simulink subsystem "quarter_car"  (R2024b)
settings: Solver=VariableStepAuto  StartTime=0.0  StopTime=10.0  RelTol=1e-3
model mask{radius=1, spin_inertia=1, offset=[0; 0; 0], ride_rate=1, damp_rate=0, C_i=0, C_a=0, min_velocity=0, initial_spin=0}
  mask prompts: radius "Wheel radius [m]"; spin_inertia "Wheel inertia [kg m²]"; offset "Resting point offset [m]"; ride_rate "Ride rate [N/m]"; damp_rate "Daming rate [N/(m/s)]"; C_i "Traction coefficient [N]"; C_a "Sideslip coefficient [N]"; min_velocity "Minimum velocity [m/s]"; initial_spin "Initial spin [rad/s]"
libraries: aerolibutil x7, matrix_library x2, simulink x1
settings Model: Creator=yevge  LastModifiedBy=yevge

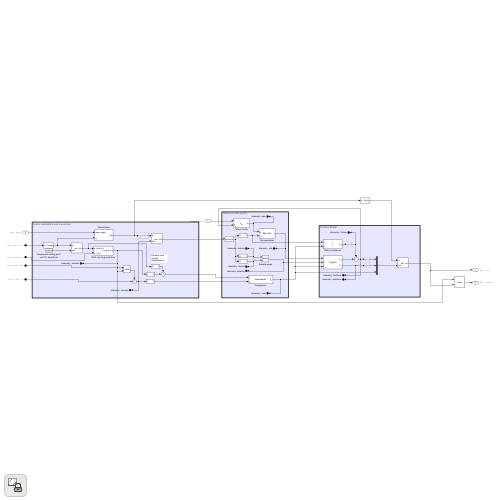
[thumbnail: Simulink's stored preview of the top-level diagram]
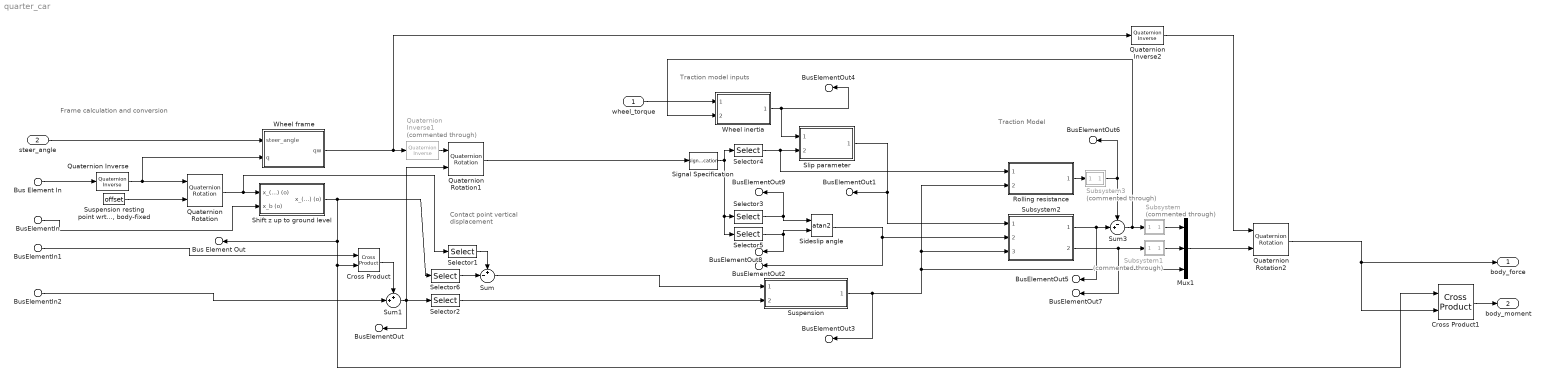
== system quarter_car ==
  note: Traction Model
  note: Traction model inputs
  note: Frame calculation and conversion
  note: Contact point vertical displacement
  wheel_torque : Inport  Unit=N*m@torque
  steer_angle : Inport  Port=2  Unit=rad
  Bus Element In : Inport  Port=3  PortName=vehicle_data  Element=ornt
  BusElementIn : Inport  Port=3  PortName=vehicle_data  Element=pos
  BusElementIn1 : Inport  Port=3  PortName=vehicle_data  Element=spin
  BusElementIn2 : Inport  Port=3  PortName=vehicle_data  Element=vel
  Cross Product : matrix_library/Cross Product
  Cross Product1 : matrix_library/Cross Product
  Mux1 : Mux  Inputs=3
  Quaternion Inverse : aerolibutil/Quaternion Inverse
  Quaternion Inverse1 : aerolibutil/Quaternion Inverse  Commented=through
  Quaternion Inverse2 : aerolibutil/Quaternion Inverse
  Quaternion Rotation : aerolibutil/Quaternion Rotation
  Quaternion Rotation1 : aerolibutil/Quaternion Rotation
  Quaternion Rotation2 : aerolibutil/Quaternion Rotation
  Rolling resistance : Subsystem  VariantControl=friction == true  ReferencedSubsystem=rolling_resistance
  Selector1 : Selector  InputPortWidth=3  IndexOptions=Index vector (dialog)  Indices=3  OutputSizes=1
  Selector2 : Selector  InputPortWidth=3  IndexOptions=Index vector (dialog)  Indices=3  OutputSizes=1
  Selector3 : Selector  InputPortWidth=3  IndexOptions=Index vector (dialog)  Indices=2  OutputSizes=1
  Selector4 : Selector  InputPortWidth=3  IndexOptions=Index vector (dialog)  Indices=1  OutputSizes=1
  Selector5 : Selector  InputPortWidth=3  IndexOptions=Index vector (dialog)  Indices=1  OutputSizes=1
  Selector6 : Selector  InputPortWidth=3  IndexOptions=Index vector (dialog)  Indices=3  OutputSizes=1
  Shift z up to ground level : Subsystem
  Sideslip angle : Trigonometry  Operator=atan2  OutputSignalType=real
  Signal Specification : SignalSpecification  Unit=m/s
  Slip parameter : Subsystem  ReferencedSubsystem=slip_model  radius=radius  min_velocity=min_velocity
  Subsystem : Subsystem  Commented=through
  Subsystem1 : Subsystem  Commented=through
  Subsystem2 : Subsystem  ReferencedSubsystem=traction  adhesion=1
  Subsystem3 : Subsystem  Commented=through
  Sum : Sum  Inputs=+-|
  Sum1 : Sum  Inputs=++|
  Sum3 : Sum  Inputs=-+|
  Suspension : Subsystem  ReferencedSubsystem=suspension  ride_rate=ride_rate  damp_rate=damp_rate
  "Suspension resting point wrt CG, body-fixed" : Constant  Value=offset
  Wheel frame : Subsystem
  Wheel inertia : Subsystem  ReferencedSubsystem=wheel_spin  radius=radius  spin_inertia=spin_inertia  initial_spin=initial_spin
  body_force : Outport  Unit=N  PortDimensions=[3 1]
  body_moment : Outport  Port=2  Unit=N*m  PortDimensions=[3 1]
  Bus Element Out : Outport  Port=3  PortName=telemetry  Element=position
  BusElementOut : Outport  Port=3  PortName=telemetry  Element=velocity
  BusElementOut1 : Outport  Port=3  PortName=telemetry  Element=slip
  BusElementOut2 : Outport  Port=3  PortName=telemetry  Element=sideslip
  BusElementOut3 : Outport  Port=3  PortName=telemetry  Element=load
  BusElementOut5 : Outport  Port=3  PortName=telemetry  Element=traction
  BusElementOut6 : Outport  Port=3  PortName=telemetry  Element=friction
  BusElementOut4 : Outport  Port=3  PortName=telemetry  Element=spin
  BusElementOut7 : Outport  Port=3  PortName=telemetry  Element=sideforce
  BusElementOut8 : Outport  Port=3  PortName=telemetry  Element=fwdvel
  BusElementOut9 : Outport  Port=3  PortName=telemetry  Element=sidevel
  wires:
  Bus Element In/1 -> Quaternion Inverse/1
  Quaternion Inverse/1 -> Wheel frame/2(q), Quaternion Rotation/1
  "Suspension resting point wrt CG, body-fixed"/1 -> Quaternion Rotation/2
  Cross Product/1 -> Sum1/1
  wheel_torque/1 -> Wheel inertia/1
  Sum1/1 -> BusElementOut/1, Selector2/1, Quaternion Rotation1/2
  Cross Product1/1 -> body_moment/1
  BusElementIn1/1 -> Cross Product/1
  BusElementIn2/1 -> Sum1/2
  Wheel inertia/1 -> BusElementOut4/1, Slip parameter/1
  Quaternion Inverse1/1 -> Quaternion Rotation1/1
  Sum/1 -> Suspension/1
  Selector2/1 -> Suspension/2
  Selector3/1 -> Sideslip angle/1, BusElementOut9/1
  Selector5/1 -> BusElementOut8/1, Sideslip angle/2
  Slip parameter/1 -> Subsystem2/1, BusElementOut1/1
  Wheel frame/1(qw) -> Quaternion Inverse1/1, Quaternion Inverse2/1
  Quaternion Rotation2/1 -> body_force/1, Cross Product1/2
  Mux1/1 -> Quaternion Rotation2/2
  Quaternion Inverse2/1 -> Quaternion Rotation2/1
  Suspension/1 -> BusElementOut3/1, Rolling resistance/2, Subsystem2/3, Mux1/3
  Subsystem/1(Out1) -> Mux1/1
  Subsystem1/1(Out1) -> Mux1/2
  Quaternion Rotation1/1 -> Signal Specification/1
  Sum3/1 -> Subsystem/1(fwd_force), Wheel inertia/2
  Rolling resistance/1 -> Subsystem3/1(fwd_force)
  Selector4/1 -> Slip parameter/2, Rolling resistance/1
  Subsystem2/1 -> Sum3/2, BusElementOut5/1
  Subsystem2/2 -> Subsystem1/1(fwd_force), BusElementOut7/1
  Subsystem3/1(Out1) -> Sum3/1, BusElementOut6/1
  Signal Specification/1 -> Selector4/1, Selector5/1, Selector3/1
  Sideslip angle/1 -> Subsystem2/2, BusElementOut2/1
  Quaternion Rotation/1 -> Shift z up to ground level/1(x_(w/b) (o)), Selector1/1
  BusElementIn/1 -> Shift z up to ground level/2(x_b (o))
  Shift z up to ground level/1(x_(cp/b) (o)) -> Selector6/1, Bus Element Out/1, Cross Product/2, Cross Product1/1
  Selector1/1 -> Sum/1
  Selector6/1 -> Sum/2
  steer_angle/1 -> Wheel frame/1(steer_angle)

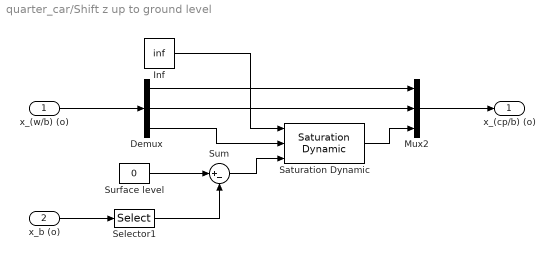
== system quarter_car/Shift z up to ground level ==
  x_(w/b) (o) : Inport
  x_b (o) : Inport  Port=2
  Demux : Demux  Outputs=3
  Inf : Constant  Value=inf  OutDataTypeStr=Inherit: Inherit via back propagation
  Mux2 : Mux  Inputs=3
  Saturation Dynamic : simulink/Discontinuities/Saturation Dynamic  OutMin=[]  OutMax=[]  OutDataTypeStr=Inherit: Same as second input  OutDataType=fixdt(1, 16)  OutScaling=2^-10  DoSatur=off
  Selector1 : Selector  InputPortWidth=3  IndexOptions=Index vector (dialog)  Indices=3  OutputSizes=1
  Sum : Sum  Inputs=|+-
  Surface level : Constant  Value=0
  x_(cp/b) (o) : Outport
  wires:
  x_(w/b) (o)/1 -> Demux/1
  Mux2/1 -> x_(cp/b) (o)/1
  Saturation Dynamic/1 -> Mux2/3
  Demux/1 -> Mux2/1
  x_b (o)/1 -> Selector1/1
  Inf/1 -> Saturation Dynamic/1
  Demux/2 -> Mux2/2
  Sum/1 -> Saturation Dynamic/3
  Demux/3 -> Saturation Dynamic/2
  Surface level/1 -> Sum/1
  Selector1/1 -> Sum/2

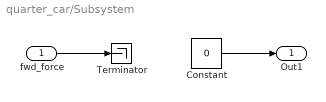
== system quarter_car/Subsystem ==
  fwd_force : Inport
  Constant : Constant  Value=0
  Terminator : Terminator
  Out1 : Outport
  wires:
  Constant/1 -> Out1/1
  fwd_force/1 -> Terminator/1

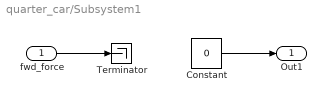
== system quarter_car/Subsystem1 ==
  fwd_force : Inport
  Constant : Constant  Value=0
  Terminator : Terminator
  Out1 : Outport
  wires:
  Constant/1 -> Out1/1
  fwd_force/1 -> Terminator/1

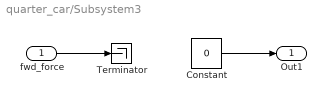
== system quarter_car/Subsystem3 ==
  fwd_force : Inport
  Constant : Constant  Value=0
  Terminator : Terminator
  Out1 : Outport
  wires:
  Constant/1 -> Out1/1
  fwd_force/1 -> Terminator/1

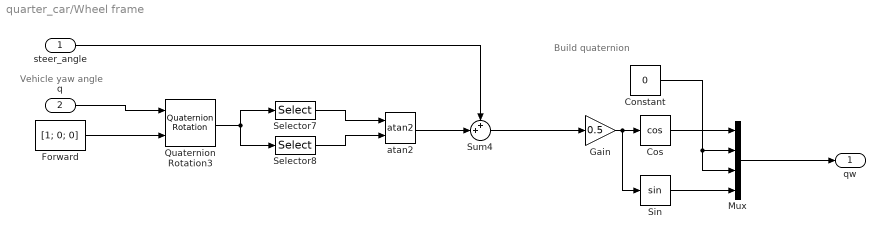
== system quarter_car/Wheel frame ==
  note: Build quaternion
  note: Vehicle yaw angle
  steer_angle : Inport  Unit=rad
  q : Inport  Port=2
  Constant : Constant  Value=0
  Cos : Trigonometry  Operator=cos
  Forward : Constant  Value=[1; 0; 0]
  Gain : Gain  Gain=0.5
  Mux : Mux
  Quaternion Rotation3 : aerolibutil/Quaternion Rotation
  Selector7 : Selector  InputPortWidth=3  IndexOptions=Index vector (dialog)  Indices=2  OutputSizes=1
  Selector8 : Selector  InputPortWidth=3  IndexOptions=Index vector (dialog)  Indices=1  OutputSizes=1
  Sin : Trigonometry
  Sum4 : Sum  Inputs=++|
  atan2 : Trigonometry  Operator=atan2  OutputSignalType=real
  qw : Outport
  wires:
  Gain/1 -> Sin/1, Cos/1
  Cos/1 -> Mux/1
  Constant/1 -> Mux/3, Mux/2
  Sin/1 -> Mux/4
  Sum4/1 -> Gain/1
  Mux/1 -> qw/1
  q/1 -> Quaternion Rotation3/1
  Selector8/1 -> atan2/2
  atan2/1 -> Sum4/2
  Selector7/1 -> atan2/1
  Forward/1 -> Quaternion Rotation3/2
  steer_angle/1 -> Sum4/1
  Quaternion Rotation3/1 -> Selector7/1, Selector8/1
